simulink model "input_delay_rise"  (Simulink 8.4)
settings: Solver=ode1  StartTime=0.0  StopTime=50  FixedStep=0.001  RelTol=1e-3
settings Model: Creator=Nitin Sharma  LastModifiedBy=rkamalapurkar
settings SolverCC: AlgebraicLoopSolver=LineSearch
settings OptimizationCC: InitFltsAndDblsToZero=on
settings DebuggingCC: SaveWithParameterizedLinksMsg=none  SignalResolutionControl=TryResolveAllWithWarning
settings GRTTargetCC: TargetFcnLib=ansi_tfl_tmw.mat

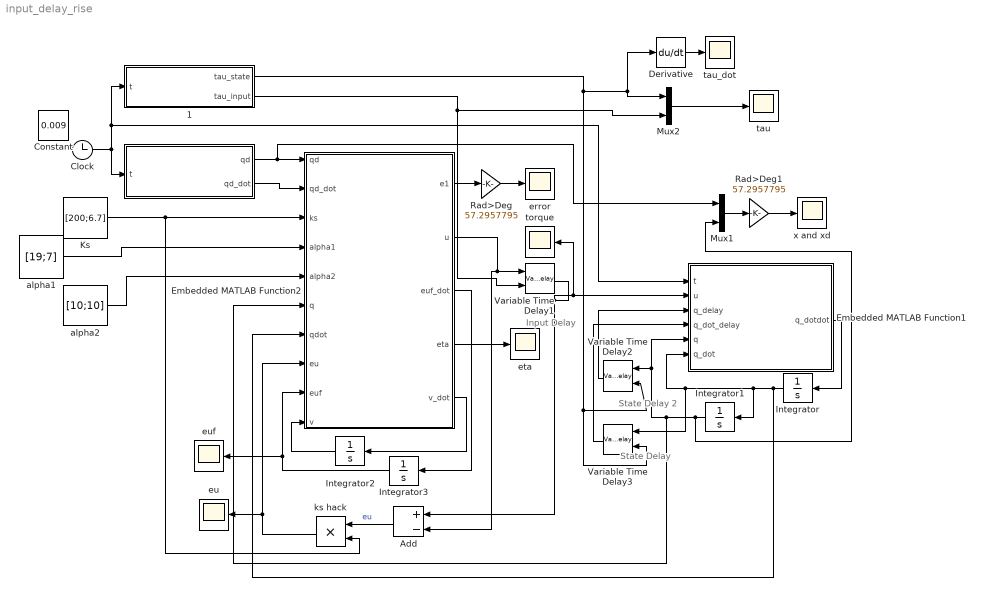
== system input_delay_rise ==
  note: State Delay 2
  note: State Delay
  note: Input Delay
  "    " : MATLAB Function  TreatAsAtomicUnit=on
  "    1" : MATLAB Function  TreatAsAtomicUnit=on
  Add : Sum  Inputs=+-
  Clock : Clock
  Derivative : Derivative
  Embedded MATLAB Function1 : MATLAB Function  TreatAsAtomicUnit=on
  Embedded MATLAB Function2 : MATLAB Function  TreatAsAtomicUnit=on
  Integrator{,1..3} (4 alike) : Integrator  InitialCondition=[0;0]
  Ks : Constant  Value=[200;6.7]
  Mux1 : Mux  Inputs=2
  Mux2 : Mux  Inputs=2
  Rad>Deg : Gain  Gain=57.2957795
  Rad>Deg1 : Gain  Gain=57.2957795
  Variable Time Delay1 : VariableTransportDelay  ZeroDelay=on
  Variable Time Delay2 : VariableTransportDelay  Tag=State Delay  ZeroDelay=on
  Variable Time Delay3 : VariableTransportDelay  Tag=State Delay  ZeroDelay=on
  alpha1 : Constant  Value=[19;7]
  alpha2 : Constant  Value=[10;10]
  error : Scope
      settings: TimeRange=50  YMin=-6  YMax=6  SaveName=error_case1
  eta : Scope
      settings: TimeRange=30  YMin=-0.4  YMax=0.4
  eu : Scope
      settings: TimeRange=50  YMin=-25  YMax=25  SaveName=ScopeData3
  euf : Scope
      settings: TimeRange=50  YMin=-2.5  YMax=2.5  SaveName=ScopeData2
  ks hack : Product  RndMeth=Zero
  tau : Scope
      settings: TimeRange=50  YMin=1.38778e-017  YMax=0.425  SaveName=tau_case1
  tau_dot : Scope
      settings: TimeRange=50  YMin=-4.853400055473372  YMax=5.122445913461537  SaveName=error2
  torque : Scope
      settings: TimeRange=50  YMin=-7  YMax=7  SaveName=u1_case1
  x and xd : Scope
      settings: TimeRange=50  YMin=-40  YMax=60  SaveName=x_xd_case1
  Constant : Constant  IOType=siggen  Value=0.009
  wires:
  Embedded MATLAB Function1/1(q_dotdot) -> Integrator/1
  Rad>Deg/1 -> error/1
  Clock/1 -> "    "/1(t), "    1"/1(t), Embedded MATLAB Function1/1(t)
  "    1"/1(tau_state) -> Mux2/1, Derivative/1, Variable Time Delay2/2, Variable Time Delay3/2
  Derivative/1 -> tau_dot/1
  "    "/1(qd) -> Embedded MATLAB Function2/1(qd), Mux1/1
  "    "/2(qd_dot) -> Embedded MATLAB Function2/2(qd_dot)
  "    1"/2(tau_input) -> Mux2/2, Variable Time Delay1/2
  Integrator2/1 -> Embedded MATLAB Function2/10(v)
  Integrator3/1 -> Embedded MATLAB Function2/9(euf), euf/1
  Variable Time Delay1/1 -> torque/1, Embedded MATLAB Function1/2(u), Add/1
  Embedded MATLAB Function2/2(u) -> Add/2, Variable Time Delay1/1
  Embedded MATLAB Function2/5(v_dot) -> Integrator2/1
  Embedded MATLAB Function2/3(euf_dot) -> Integrator3/1
  Embedded MATLAB Function2/1(e1) -> Rad>Deg/1
  ks hack/1 -> Embedded MATLAB Function2/8(eu), eu/1
  Add/1 -> ks hack/1  "eu"
  Ks/1 -> Embedded MATLAB Function2/3(ks), ks hack/2
  Mux1/1 -> Rad>Deg1/1
  Rad>Deg1/1 -> x and xd/1
  alpha1/1 -> Embedded MATLAB Function2/4(alpha1)
  alpha2/1 -> Embedded MATLAB Function2/5(alpha2)
  Embedded MATLAB Function2/4(eta) -> eta/1
  Integrator/1 -> Embedded MATLAB Function1/6(q_dot), Variable Time Delay3/1, Integrator1/1, Embedded MATLAB Function2/7(qdot)
  Integrator1/1 -> Mux1/2, Embedded MATLAB Function1/5(q), Variable Time Delay2/1, Embedded MATLAB Function2/6(q)
  Variable Time Delay2/1 -> Embedded MATLAB Function1/3(q_delay)
  Variable Time Delay3/1 -> Embedded MATLAB Function1/4(q_dot_delay)
  Mux2/1 -> tau/1

== matlab function Embedded MATLAB Function1 ==
  data: t input double; u input double; q_delay input double; q_dot_delay input double; q input double; q_dotdot output double; q_dot input double
function q_dotdot  = dynamics(t,u,q_delay,q_dot_delay,q,q_dot)

p1=3.473;
p2=.193;
p3=.242;
p4=0.467;
p5=0.234;
fd1=5.3;
fd2=1.1;
M  = [ p1+2*p3*cos(q(2))   , p2+p3*cos(q(2));
       p2+p3*cos(q(2))     , p2              ];
Vm = [ -p3*sin(q_delay(2))*q_dot_delay(2)  , -p3*sin(q_delay(2))*(q_dot_delay(1)+q_dot_delay(2));
        p3*sin(q_delay(2))*q_dot_delay(1)  , 0                                 ];
Fd = diag([fd1,fd2]);
f = [-p4*sin(q(2));
     p5*sin(q(2))*q_dot(2)];
Td = [ 0.2*sin(t/2) ; 0.1*sin(t/4) ];

%T = u - Vm*q_dot - Fd*q_dot;
T = u - Vm*q_dot_delay - Fd*q_dot_delay - f - Td;
q_dotdot=M\T;

end

== matlab function Embedded MATLAB Function2 ==
  data: qd input double; qd_dot input double; ks input double; alpha1 input double; alpha2 input double; q input double; e1 output double; u output double; qdot input double; eu input double; euf input double; v input double; euf_dot output double; eta output double; v_dot output double
function [e1,u,euf_dot,eta,v_dot] = controller(qd,qd_dot,ks,alpha1,alpha2,q,qdot,eu,euf,v)

    % time delay changes 
    %k = diag([17,0.65]); alpha1 = diag([15,32]); % slow, large
    %k = diag([80,15]); alpha1 = diag([35,25]); % slow, small
    %k = diag([15,0.9]); alpha1 = diag([20,29]); % fast, large
    %k = diag([80,15]); alpha1 = diag([35,25]); % fast, small
    
    alpha1_d = diag(alpha1); 
    alpha2_d = diag(alpha2);
    ks_d = diag(ks);
    
    % Proposed
    e1 = qd - q;
    e1_dot = qd_dot - qdot; 
    e2 = e1_dot + alpha1_d*e1;
    euf_dot = -alpha2_d*euf + eu;
    eta = e2+euf;
    u = ks_d*e2 + v;
    v_dot = ks_d*e2 + eu;% + beta_d*sign(eta);  % eu is already multiplied by ks outside the controller block
    
end


% 0 delay:
% ks=65,3.5
% a1=65,25
% a2=200,20
% beta=1,0.2

== matlab function     1 ==
  data: tau_state output double; t input double; tau_input output double
function [tau_state,tau_input] = TimeDelay(t)

% test1 -- input: slow, large
% magVal_i = 0.05; phaseVal_i = 10; offset_i = 0.1; %input - slow, large 
% magVal_s = 0.005; phaseVal_s = 8; offset_s = 0.01; %state - slow, small
% % 250,1.83 | 19.5,7.5 | 1.5,1.5 |error<3 degree

% test2 -- input: fast, small
% magVal_i = 0.01; phaseVal_i = 3; offset_i = 0.03; %input - fast, small
% magVal_s = 0.01; phaseVal_s = 2; offset_s = 0.04; %state - fast, large
% % 200,4.6 | 15,8 | 10,10 |error<0.92 degree
% 
% % test3 -- input: fast, large
% magVal_i = 0.05; phaseVal_i = 2; offset_i = 0.1; %input - fast, large
% magVal_s = 0.01; phaseVal_s = 10; offset_s = 0.04; %state - slow, large
% 200,1.5 | 19.5,7.5 | 10,10 |error<3.57 degree

% % test4 -- input: slow, large
% magVal_i = 0.05; phaseVal_i = 10; offset_i = 0.1; %input - slow, large
% magVal_s = 0.01; phaseVal_s = 10; offset_s = 0.04; %state - slow, large
% 100,1.33 | 19,7 | 10,10 |error<4.21 degree

% % % test5 -- 
magVal_i = 0.005; phaseVal_i = 2; offset_i = 0.03; %input - fast, small
magVal_s = 0.05; phaseVal_s = 1; offset_s = .8; %state - fast, large
% 200,6.7 | 19,7 | 10,10 |error<0.7 degree

% test4 compare to UUB
%  magVal_i = 0.01; phaseVal_i = 3; offset_i = 0.03; %input - fast, small
%  magVal_s = 0; phaseVal_s = 2; offset_s = 0; %state - fast, large
% 200,6.7 | 19,7 | 10,10 | error<0.76 degree


% input delay
%magVal_i = 0.02; phaseVal_i = 10; offset_i = 0.03;
tau_input = magVal_i*sin(t/phaseVal_i)+offset_i;

% state delay
%magVal_s = 0.001; phaseVal_s = 3; offset_s = 0.005;
tau_state = magVal_s*sin(t/phaseVal_s)+offset_s;

% good gains
% 80,2.5
% 30,13
% 100,10
% 0.7,0.1

end

== matlab function      ==
  data: qd output double; qd_dot output double; t input double
function [qd,qd_dot] = TrajGen(t)

qd = [(30*(3.1415/180)*sin(1.5*t)+20*(3.1415/180))*(1-exp(-0.01*t^3)); -(20*(3.1415/180)*sin(0.5*t)+10*(3.1415/180))*(1-exp(-0.01*t^3))];
qd_dot = [    (3*t^2*((6283*sin((3*t)/2))/12000 + 6283/18000))/(100*exp(t^3/100)) - (6283*cos((3*t)/2)*(1/exp(t^3/100) - 1))/8000;
        (6283*cos(t/2)*(1/exp(t^3/100) - 1))/36000 - (3*t^2*((6283*sin(t/2))/18000 + 6283/36000))/(100*exp(t^3/100)) ];

% qd = [0.1*sin(t);0.5*sin(t)];
% qd_dot = [0.1*cos(t);0.5*cos(t)];

end
